simulink model "Miss_Sim_MatrixPilot"  (Simulink 7.0)
settings: Solver=ode1  SolverMode=SingleTasking  StartTime=0.0  StopTime=120  FixedStep=0.00025  MaxStep=0.01  MinStep=0.000001  RelTol=1e-12  AbsTol=1e-12
values from neighbouring files (symbols this model uses):
  alpha = [-180.     -90.        -5.         0.         5.        10.        15.        90.       180.       ]    [Miss_Data.m]
  Bref = 1.4    [Miss_Data.m]
  Clail = [ 0.         0.         0.         0.         0.         0.         0.         0.         0.       ]    [Miss_Data.m]
  Clp = [-0.5000    -0.5000    -0.496303  -0.494610  -0.492441  -0.492625  -0.522141  -0.5000    -0.5000   ]    [Miss_Data.m]
  Clr = [ 0.         0.         0.064175   0.123689   0.182593   0.241565   0.304725   0.         0.       ]    [Miss_Data.m]
  Clrud = [-0.000045  -0.000045  -0.000051  -0.000049  -0.000047  -0.000043  -0.000039  -0.000045  -0.000045 ]    [Miss_Data.m]
  Clv = [ 0.         0.        -0.098934  -0.137639  -0.176627  -0.217863  -0.281334   0.         0.       ]    [Miss_Data.m]
  Cmele = [-0.0180    -0.0180    -0.019125  -0.019236  -0.019052  -0.018576  -0.017796  -0.0180    -0.0180   ]    [Miss_Data.m]
  Cmq = [-12.3     -12.3      -12.288971 -12.358734 -12.331396 -12.223111 -12.072741 -12.3      -12.3      ]    [Miss_Data.m]
  Cmtot = [ 0.         2.         0.097340   0.036740  -0.047230  -0.137480  -0.110880  -2.         0.       ]    [Miss_Data.m]
  Cnail = [ 0.         0.         0.         0.         0.         0.         0.         0.         0.       ]    [Miss_Data.m]
  Cnp = [ 0.         0.         0.027830  -0.031473  -0.087981  -0.137950  -0.158851   0.         0.       ]    [Miss_Data.m]
  Cnr = [ 0.         0.        -0.041684  -0.040009  -0.043373  -0.056062  -0.120565   0.         0.       ]    [Miss_Data.m]
  Cnrud = [ 0.         0.         0.000628   0.000668   0.000698   0.000717   0.000725   0.         0.       ]    [Miss_Data.m]
  Cnv = [ 0.         0.         0.011072   0.000612  -0.009401  -0.018785  -0.019172   0.         0.       ]    [Miss_Data.m]
  Cref = 0.20    (= 0.2)    [Miss_Data.m]
  CROSS_TRACK = 1    [MatrixPilot_Parameters.m]
  CXq = [ 0.         0.        -0.507981  -0.147630   0.201483   0.570203   1.026474   0.         0.       ]    [Miss_Data.m]
  CXtot = [ 0.03       0.        -0.060470  -0.054540   0.003010   0.075240  -0.109550   0.         0.03     ]    [Miss_Data.m]
  CYp = [ 0.         0.        -0.217329  -0.145848  -0.074905  -0.009210   0.015572   0.         0.       ]    [Miss_Data.m]
  CYr = [ 0.         0.         0.049134   0.076782   0.103755   0.129584   0.152004   0.         0.       ]    [Miss_Data.m]
  CYrud = [-0.0016    -0.0016    -0.001484  -0.001575  -0.001641  -0.001681  -0.001693  -0.0016    -0.0016   ]    [Miss_Data.m]
  CYv = [ 0.         0.        -0.204296  -0.201289  -0.208918  -0.263073  -0.644029   0.         0.       ]    [Miss_Data.m]
  CZele = [-0.0067    -0.0067    -0.006924  -0.006962  -0.006897  -0.006734  -0.006498  -0.0067    -0.0067   ]    [Miss_Data.m]
  CZq = [ 0.         0.        -9.116849  -8.745556  -8.332987  -7.894125  -7.541102   0.         0.       ]    [Miss_Data.m]
  CZtot = [ 0.        10.         0.102580  -0.382550  -0.864940  -1.339340  -1.876430 -10.         0.       ]    [Miss_Data.m]
  DH = 10.    (= 10)    [MatrixPilot_Parameters.m]
  ele_damping = 0.7    [Miss_Data.m]
  ele_def_max = 30.    (= 30)    [Miss_Data.m]
  ele_frequency = 150.    (= 150)    [Miss_Data.m]
  ele_rate_limit = 285.    (= 285)    [Miss_Data.m]
  Ixx = 0.03004    [Miss_Data.m]
  Ixy = 0.    (= 0)    [Miss_Data.m]
  Ixz = 0.00137    [Miss_Data.m]
  Iyx = Ixy    (= 0)    [Miss_Data.m]
  Iyy = 0.01916    [Miss_Data.m]
  Iyz = 0.    (= 0)    [Miss_Data.m]
  Izx = Ixz    (= 0.00137)    [Miss_Data.m]
  Izy = Iyz    (= 0)    [Miss_Data.m]
  Izz = 0.04573    [Miss_Data.m]
  Mass = 0.950    (= 0.95)    [Miss_Data.m]
  rud_damping = 0.7    [Miss_Data.m]
  rud_def_max = 30.    (= 30)    [Miss_Data.m]
  rud_frequency = 150.    (= 150)    [Miss_Data.m]
  rud_rate_limit = 285.    (= 285)    [Miss_Data.m]
  SPEED_CONTROL = 1    [MatrixPilot_Parameters.m]
  Sref = 0.28    [Miss_Data.m]
  T_max = 1.    (= 1)    [MatrixPilot_Parameters.m]
  T_min = 0.35    [MatrixPilot_Parameters.m]
  Tdgps = 1.    (= 1)    [Miss_Data.m]
  theta_0 = -15.    (= -15)    [MatrixPilot_Parameters.m]
  theta_max = 15.    (= 15)    [MatrixPilot_Parameters.m]
  theta_min = -15.    (= -15)    [MatrixPilot_Parameters.m]
  Tmax = 10.    (= 10)    [Miss_Data.m]
  Vsp = 10.    (= 10)    [MatrixPilot_Parameters.m]
  WAYPOINT_RADIUS = 30.    (= 30)    [MatrixPilot_Parameters.m]
undefined symbols (not defined in the file or in its folder): F, MIL, Moderate
libraries: simulink x41, simulink_extras x26, dspstat3 x2, aerospace x1, aerolibanim x1, aerolibwind2 x1
(part 1 of 2)
settings Model: Creator=bizard  LastModifiedBy=bizard
settings SolverCC: InitialStep=0.000001  AutoInsertRateTranBlk=on
settings OptimizationCC: BooleanDataType=off
settings DebuggingCC: SaveWithParameterizedLinksMsg=none  SignalResolutionControl=TryResolveAllWithWarning  SolverPrmCheckMsg=none  MultiTaskDSMMsg=warning  MultiTaskCondExecSysMsg=none  StrictBusMsg=None
settings HardwareCC: TargetEndianess=LittleEndian  TargetHWDeviceType=MATLAB Host  ProdEqTarget=off
settings RTWCC: IncludeERTFirstTime=on

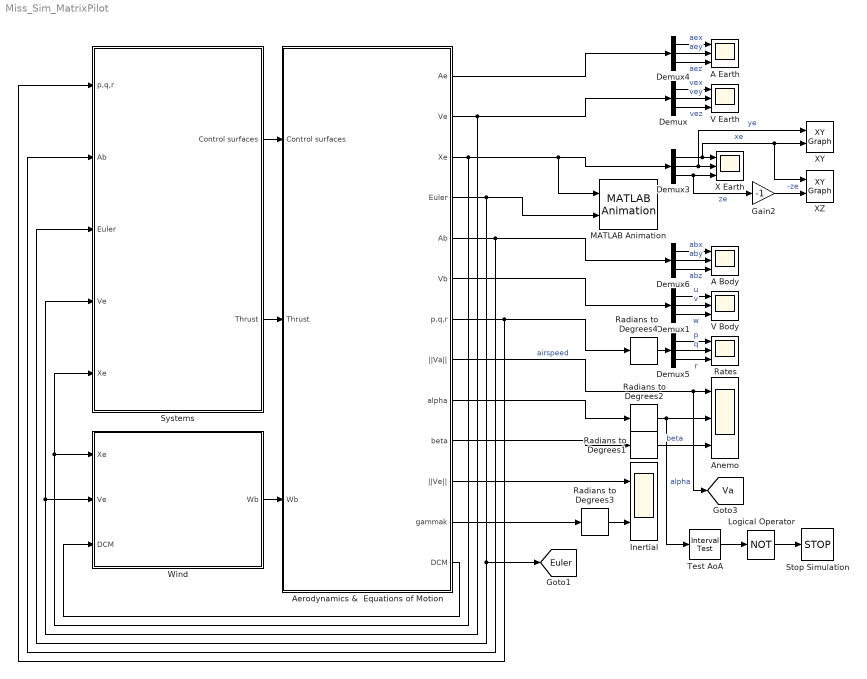
== system Miss_Sim_MatrixPilot ==
  A Body : Scope  NumInputPorts=3
      settings: TimeRange=300  YMin=0~-0.1~0  YMax=30~0.1~2  SaveName=ScopeData3  MaxDataPoints=60000  Decimation=10
  A Earth : Scope  NumInputPorts=3
      settings: TimeRange=60  YMin=-10~-10~-4  YMax=10~10~8  MaxDataPoints=600000  Decimation=10
  Aerodynamics &  Equations of Motion : Subsystem
  Anemo : Scope  NumInputPorts=3
      settings: TimeRange=20  YMin=8.7~0~-8  YMax=10.3~5~8  SaveName=ScopeData6  MaxDataPoints=600000  Decimation=10
  Demux{,1,3..6} (6 alike) : Demux  Outputs=3
  Gain2 : Gain  Gain=-1  SaturateOnIntegerOverflow=on
  Inertial : Scope  NumInputPorts=2
      settings: TimeRange=50  YMin=7.5~-10  YMax=10.5~-0  SaveName=ScopeData7  MaxDataPoints=600000  Decimation=10
  Logical Operator : Logic  Operator=NOT  AllPortsSameDT=off  OutDataTypeMode=boolean
  MATLAB Animation : aerolibanim/MATLAB Animation  Vehicles=1  Geometries='astredwedge.mat'  BoundingBoxCoordinates=[-50,50,-50,50,-50,50]  CameraOffset=[-150,-50,0]  CameraViewAngle=3  SampleTime=0.1  FigurePosition=[1080,494,275,214]
  Radians to Degrees{1..4} (4 alike) : simulink_extras/Transformations/Radians to Degrees  SystemSampleTime=-1
  Rates : Scope  NumInputPorts=3
      settings: YMin=-100~-100~-100  YMax=100~100~100  MaxDataPoints=600000  Decimation=10
  Stop Simulation : Stop
  Systems : Subsystem
  Test AoA : simulink/Logic and Bit Operations/Interval Test  SystemSampleTime=-1  IntervalClosedRight=on  uplimit=15  IntervalClosedLeft=on  lowlimit=-15  LogicOutDataTypeMode=boolean
  V Body : Scope  NumInputPorts=3
      settings: TimeRange=300  YMin=0~-0.1~0  YMax=30~0.1~2  SaveName=ScopeData4  MaxDataPoints=60000  Decimation=10
  V Earth : Scope  NumInputPorts=3
      settings: TimeRange=60  YMin=-15~-15~-3  YMax=10~15~2  SaveName=ScopeData2  MaxDataPoints=600000  Decimation=10  SampleInput=on
  Wind : Subsystem
  X Earth : Scope  NumInputPorts=3
      settings: TimeRange=60  YMin=-150~-100~-80  YMax=150~100~-45  SaveName=ScopeData9  MaxDataPoints=600000  Decimation=10
  XY : simulink/Sinks/XY Graph  SystemSampleTime=-1  xmin=-150  xmax=150  ymin=-150  ymax=150  st=.1
  XZ : simulink/Sinks/XY Graph  SystemSampleTime=-1  xmin=-150  xmax=150  ymin=0  ymax=100  st=.1
  tag scope: Euler=global, Va=global
  wires:
  Aerodynamics &  Equations of Motion/9(alpha) -> Radians to Degrees2/1
  Aerodynamics &  Equations of Motion/10(beta) -> Radians to Degrees1/1
  Radians to Degrees1/1 -> Anemo/3  "beta"
  Demux1/1 -> V Body/1  "u"
  Demux1/2 -> V Body/2  "v"
  Demux1/3 -> V Body/3  "w"
  Radians to Degrees2/1 -> Anemo/2, Test AoA/1  "alpha"
  Aerodynamics &  Equations of Motion/8(||Va||) -> Anemo/1, [Va]  "airspeed"
  Demux5/1 -> Rates/1  "p"
  Demux5/2 -> Rates/2  "q"
  Demux5/3 -> Rates/3  "r"
  Radians to Degrees4/1 -> Demux5/1
  Aerodynamics &  Equations of Motion/7(p,q,r) -> Radians to Degrees4/1, Systems/1(p,q,r)
  Aerodynamics &  Equations of Motion/6(Vb) -> Demux1/1
  Aerodynamics &  Equations of Motion/4(Euler) -> MATLAB Animation/2, Systems/3(Euler), [Euler]
  Demux/1 -> V Earth/1  "vex"
  Demux/2 -> V Earth/2  "vey"
  Demux/3 -> V Earth/3  "vez"
  Gain2/1 -> XZ/2  "-ze"
  Aerodynamics &  Equations of Motion/3(Xe) -> Demux3/1, MATLAB Animation/1, Systems/5(Xe), Wind/1(Xe)
  Aerodynamics &  Equations of Motion/2(Ve) -> Systems/4(Ve), Wind/2(Ve), Demux/1
  Systems/2(Thrust) -> Aerodynamics &  Equations of Motion/2(Thrust)
  Systems/1(Control surfaces) -> Aerodynamics &  Equations of Motion/1(Control surfaces)
  Aerodynamics &  Equations of Motion/1(Ae) -> Demux4/1
  Demux4/3 -> A Earth/3  "aez"
  Demux4/2 -> A Earth/2  "aey"
  Demux4/1 -> A Earth/1  "aex"
  Demux6/1 -> A Body/1  "abx"
  Demux6/3 -> A Body/3  "abz"
  Aerodynamics &  Equations of Motion/5(Ab) -> Demux6/1, Systems/2(Ab)
  Wind/1(Wb) -> Aerodynamics &  Equations of Motion/3(Wb)
  Demux6/2 -> A Body/2  "aby"
  Test AoA/1 -> Logical Operator/1
  Logical Operator/1 -> Stop Simulation/1
  Aerodynamics &  Equations of Motion/11(||Ve||) -> Inertial/1
  Aerodynamics &  Equations of Motion/13(DCM) -> Wind/3(DCM)
  Demux3/1 -> X Earth/1, XY/2, XZ/1  "xe"
  Demux3/2 -> X Earth/2, XY/1  "ye"
  Demux3/3 -> X Earth/3, Gain2/1  "ze"
  Aerodynamics &  Equations of Motion/12(gammak) -> Radians to Degrees3/1
  Radians to Degrees3/1 -> Inertial/2

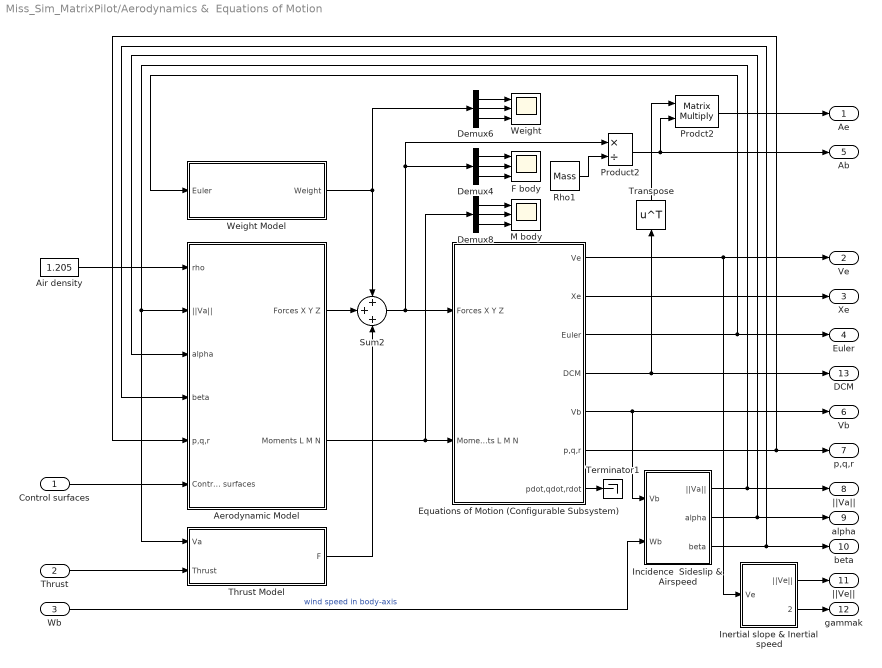
== system Miss_Sim_MatrixPilot/Aerodynamics &  Equations of Motion ==
  Control surfaces : Inport
  Thrust : Inport  Port=2
  Wb : Inport  Port=3
  Aerodynamic Model : Subsystem
  Air density : Constant  Value=1.205
  Demux4 : Demux  Outputs=3
  Demux6 : Demux  Outputs=3
  Demux8 : Demux  Outputs=3
  Equations of Motion (Configurable Subsystem) : Subsystem  BlockChoice=Quaternions
      link override Euler Angles: Inertia=[Ixx Ixy Ixz ; Iyx Iyy Iyz ; Izx Izy Izz]  eul_0="[0.    0.    0.]"  Vm_0="[25.   0.   0.]"  Mass=Mass  xme_0=[0. 0. 0.]
      link override Quaternions: Inertia="[Ixx  -Ixy  -Ixz;  -Iyx  Iyy  -Iyz;  -Izx  -Izy  Izz]"  Mass=Mass  Vm_0=[10 0 0]  eul_0=[0 0. 0]  xme_0=[0 0 -75.]
      settings: AttributesFormatString=%<BlockChoice>  MemberBlocks=Euler Angles,Quaternions
      settings: TemplateBlock=|
      | aerospace/6DoF/Equations of Motion
      | (Configurable Subsystem)
  F body : Scope  NumInputPorts=3
      settings: YMin=-20~-1~-100  YMax=27.5~1~10  SaveName=ScopeData5  MaxDataPoints=600000  Decimation=10
  Incidence  Sideslip & Airspeed : Subsystem
  Inertial slope & Inertial speed : Subsystem
  M body : Scope  NumInputPorts=3
      settings: TimeRange=300  YMin=13~-1~-2.5  YMax=20.5~1~1.5  SaveName=ScopeData10  MaxDataPoints=600000  Decimation=10
  Prodct2 : Product  Multiplication=Matrix(*)  SaturateOnIntegerOverflow=on  RndMeth=Zero  InputSameDT=on
  Product2 : Product  Inputs=*/  SaturateOnIntegerOverflow=on  RndMeth=Zero  InputSameDT=on
  Rho1 : Constant  Value=Mass
  Sum2 : Sum  Inputs=+++  SaturateOnIntegerOverflow=on  InputSameDT=on
  Terminator1 : Terminator
  Thrust Model : Subsystem
  Transpose : Math  Orientation=up  Operator=transpose  SaturateOnIntegerOverflow=on
  "Weight " : Scope  NumInputPorts=3
      settings: TimeRange=300  YMin=13~-1~0  YMax=20.5~1~50  SaveName=ScopeData8  MaxDataPoints=600000  Decimation=10
  Weight Model : Subsystem
  Ae : Outport
  Ve : Outport  Port=2
  Xe : Outport  Port=3
  Euler : Outport  Port=4
  Ab : Outport  Port=5
  Vb : Outport  Port=6
  p,q,r : Outport  Port=7
  ||Va|| : Outport  Port=8
  alpha : Outport  Port=9
  beta : Outport  Port=10
  ||Ve|| : Outport  Port=11
  gammak : Outport  Port=12
  DCM : Outport  Port=13
  wires:
  Equations of Motion (Configurable Subsystem)/7(pdot,qdot,rdot) -> Terminator1/1
  Equations of Motion (Configurable Subsystem)/1(Ve) -> Inertial slope & Inertial speed/1(Ve), Ve/1
  Equations of Motion (Configurable Subsystem)/3(Euler) -> Weight Model/1(Euler), Euler/1
  Equations of Motion (Configurable Subsystem)/5(Vb) -> Incidence  Sideslip & Airspeed/1(Vb), Vb/1
  Incidence  Sideslip & Airspeed/2(alpha) -> alpha/1, Aerodynamic Model/3(alpha)
  Equations of Motion (Configurable Subsystem)/6(p,q,r) -> p,q,r/1, Aerodynamic Model/5(p,q,r)
  Incidence  Sideslip & Airspeed/3(beta) -> beta/1, Aerodynamic Model/4(beta)
  Incidence  Sideslip & Airspeed/1(||Va||) -> ||Va||/1, Aerodynamic Model/2(||Va||), Thrust Model/1(Va)
  Equations of Motion (Configurable Subsystem)/2(Xe) -> Xe/1
  Thrust Model/1(F) -> Sum2/3
  Weight Model/1(Weight) -> Sum2/1, Demux6/1
  Demux4/1 -> F body/1
  Demux4/2 -> F body/2
  Demux4/3 -> F body/3
  Aerodynamic Model/1(Forces X Y Z) -> Sum2/2
  Sum2/1 -> Equations of Motion (Configurable Subsystem)/1(Forces X Y Z), Demux4/1, Product2/1
  Inertial slope & Inertial speed/1(||Ve||) -> ||Ve||/1
  Inertial slope & Inertial speed/2(gammak) -> gammak/1
  Demux6/1 -> "Weight "/1
  Demux6/2 -> "Weight "/2
  Demux6/3 -> "Weight "/3
  Demux8/1 -> M body/1
  Demux8/2 -> M body/2
  Demux8/3 -> M body/3
  Aerodynamic Model/2(Moments L M N) -> Demux8/1, Equations of Motion (Configurable Subsystem)/2(Moments L M N)
  Control surfaces/1 -> Aerodynamic Model/6(Control surfaces)
  Thrust/1 -> Thrust Model/2(Thrust)
  Product2/1 -> Ab/1, Prodct2/2
  Equations of Motion (Configurable Subsystem)/4(DCM) -> Transpose/1, DCM/1
  Transpose/1 -> Prodct2/1
  Prodct2/1 -> Ae/1
  Wb/1 -> Incidence  Sideslip & Airspeed/2(Wb)  "wind speed in body-axis"
  Rho1/1 -> Product2/2
  Air density/1 -> Aerodynamic Model/1(rho)

== system Miss_Sim_MatrixPilot/Systems ==
  p,q,r : Inport
  Ab : Inport  Port=2
  Euler : Inport  Port=3
  Ve : Inport  Port=4
  Xe : Inport  Port=5
  Actuators : Subsystem
  Data processing : Subsystem
  NGC : Subsystem
  Sensors : Subsystem
  Control surfaces : Outport
  Thrust : Outport  Port=2
  wires:
  NGC/1(rudc) -> Actuators/1(rudc)
  NGC/2(elec) -> Actuators/2(elec)
  Actuators/1(Control surfaces) -> Control surfaces/1
  Actuators/2(Thrust) -> Thrust/1
  NGC/3(Tc) -> Actuators/3(Tc)
  p,q,r/1 -> Sensors/1(p,q,r)
  Xe/1 -> Sensors/5(Xe)
  Ve/1 -> Sensors/4(Ve)
  Euler/1 -> Sensors/3(Euler)
  Ab/1 -> Sensors/2(Ab)
  Data processing/4(||Va||) -> NGC/4(||Va||)
  Data processing/1(DCM) -> NGC/1(DCM)
  Data processing/2(We) -> NGC/2(We)
  Sensors/2(GPS) -> Data processing/2(GPS)
  Data processing/3(Vaxy) -> NGC/3(Vaxy)
  Sensors/1(Acc) -> Data processing/1(Acc)
  Sensors/3("p,q,r ") -> Data processing/3(p,q,r), NGC/7(p,q,r)
  Data processing/6(Ve) -> NGC/6(Ve)
  Data processing/5(Xe) -> NGC/5(Xe)

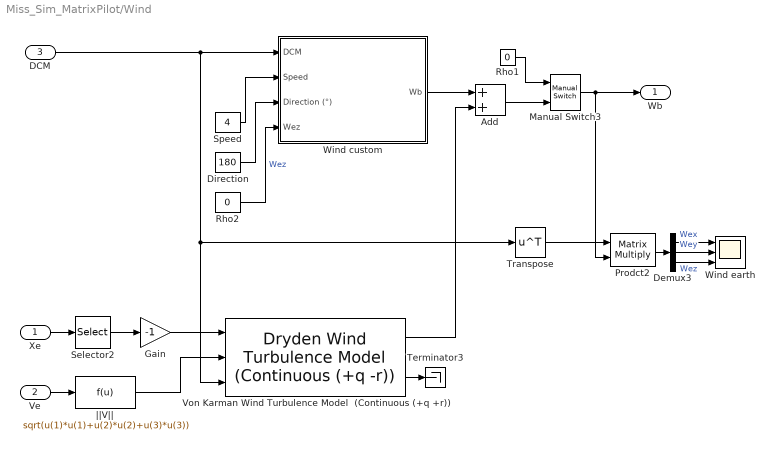
== system Miss_Sim_MatrixPilot/Wind ==
  Xe : Inport
  Ve : Inport  Port=2
  DCM : Inport  Port=3
  Add : Sum  OutDataType=sfix(16)  OutScaling=2^-10
  Demux3 : Demux  Outputs=3
  Direction : Constant  Value=180
  Gain : Gain  Gain=-1  ParameterDataType=sfix(16)  ParameterScaling=2^0  OutDataType=sfix(16)  OutScaling=2^0
  Manual Switch3 : simulink/Signal Routing/Manual Switch  SystemSampleTime=-1  sw=1  action=0  varsize=off
  Prodct2 : Product  Multiplication=Matrix(*)  SaturateOnIntegerOverflow=on  RndMeth=Zero  InputSameDT=on
  Rho1 : Constant  Value=0  VectorParams1D=off
  Rho2 : Constant  Value=0
  Selector2 : Selector  InputPortWidth=3  IndexOptions=Index vector (dialog)  Indices=[3]  OutputSizes=1
  Speed : Constant  Value=4
  Terminator3 : Terminator
  Transpose : Math  Operator=transpose  SaturateOnIntegerOverflow=on
  Von Karman Wind Turbulence Model  (Continuous (+q +r)) : aerolibwind2/Dryden Wind Turbulence Model  (Continuous (+q -r))  SystemSampleTime=-1  units=Metric (MKS)  spec=MIL-F-8785C  model=Continuous Dryden (-q +r)  W20=4  Wdeg=180  TurbProb=10^-3 - Moderate  L_high=762  Wingspan=1.4  ts=1  Seed=[23341 23342 23343 23344]  T_on=on
  Wind custom : Subsystem
  Wind earth : Scope  NumInputPorts=3
      settings: TimeRange=60  YMin=-1~-1~-1  YMax=1~1~1  SaveName=ScopeData33  MaxDataPoints=600000  Decimation=100
  ||V|| : Fcn  Expr=sqrt(u(1)*u(1)+u(2)*u(2)+u(3)*u(3))
  Wb : Outport
  wires:
  Direction/1 -> Wind custom/3(Direction (°))
  Speed/1 -> Wind custom/2(Speed)
  Rho2/1 -> Wind custom/4(Wez)  "Wez"
  DCM/1 -> Wind custom/1(DCM), Von Karman Wind Turbulence Model  (Continuous (+q +r))/3, Transpose/1
  Ve/1 -> ||V||/1
  Xe/1 -> Selector2/1
  ||V||/1 -> Von Karman Wind Turbulence Model  (Continuous (+q +r))/2
  Gain/1 -> Von Karman Wind Turbulence Model  (Continuous (+q +r))/1
  Wind custom/1(Wb) -> Add/1
  Add/1 -> Manual Switch3/2
  Von Karman Wind Turbulence Model  (Continuous (+q +r))/1 -> Add/2
  Von Karman Wind Turbulence Model  (Continuous (+q +r))/2 -> Terminator3/1
  Demux3/1 -> Wind earth/1  "Wex"
  Demux3/2 -> Wind earth/2  "Wey"
  Demux3/3 -> Wind earth/3  "Wez"
  Prodct2/1 -> Demux3/1
  Transpose/1 -> Prodct2/1
  Rho1/1 -> Manual Switch3/1
  Manual Switch3/1 -> Wb/1, Prodct2/2
  Selector2/1 -> Gain/1

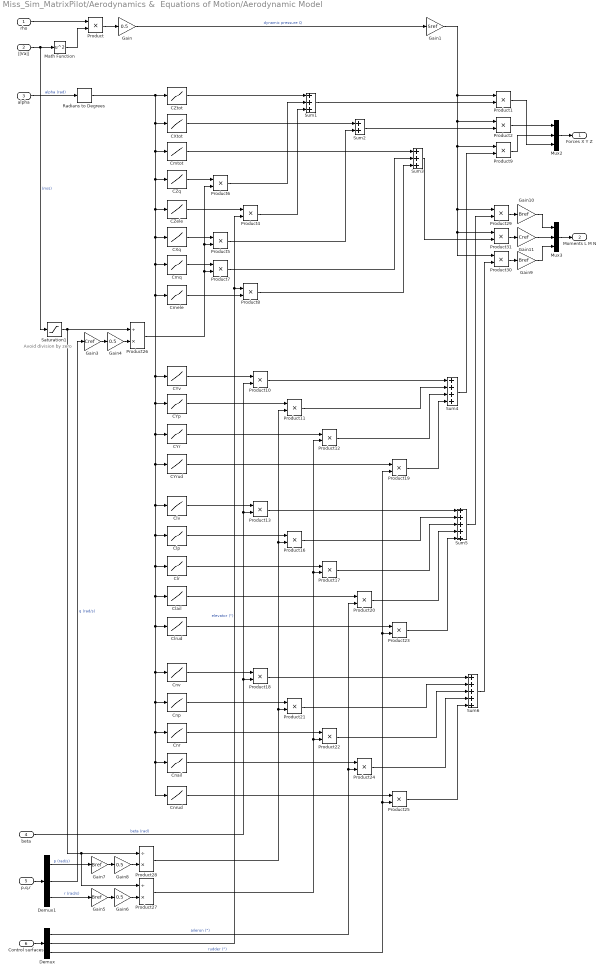
== system Miss_Sim_MatrixPilot/Aerodynamics &  Equations of Motion/Aerodynamic Model ==
  note: Avoid division
      | by zero
  rho : Inport
  ||Va|| : Inport  Port=2
  alpha : Inport  Port=3
  beta : Inport  Port=4
  p,q,r : Inport  Port=5
  Control surfaces : Inport  Port=6
  CXq : Lookup  InputValues=alpha  Table=CXq  SaturateOnIntegerOverflow=on
  CXtot : Lookup  InputValues=alpha  Table=CXtot  SaturateOnIntegerOverflow=on
  CYp : Lookup  InputValues=alpha  Table=CYp  SaturateOnIntegerOverflow=on
  CYr : Lookup  InputValues=alpha  Table=CYr  SaturateOnIntegerOverflow=on
  CYrud : Lookup  InputValues=alpha  Table=CYrud  SaturateOnIntegerOverflow=on
  CYv : Lookup  InputValues=alpha  Table=CYv  SaturateOnIntegerOverflow=on
  CZele : Lookup  InputValues=alpha  Table=CZele  SaturateOnIntegerOverflow=on
  CZq : Lookup  InputValues=alpha  Table=CZq  SaturateOnIntegerOverflow=on
  CZtot : Lookup  InputValues=alpha  Table=CZtot  SaturateOnIntegerOverflow=on
  Clail : Lookup  InputValues=alpha  Table=Clail  SaturateOnIntegerOverflow=on
  Clp : Lookup  InputValues=alpha  Table=Clp  SaturateOnIntegerOverflow=on
  Clr : Lookup  InputValues=alpha  Table=Clr  SaturateOnIntegerOverflow=on
  Clrud : Lookup  InputValues=alpha  Table=Clrud  SaturateOnIntegerOverflow=on
  Clv : Lookup  InputValues=alpha  Table=Clv  SaturateOnIntegerOverflow=on
  Cmele : Lookup  InputValues=alpha  Table=Cmele  SaturateOnIntegerOverflow=on
  Cmq : Lookup  InputValues=alpha  Table=Cmq  SaturateOnIntegerOverflow=on
  Cmtot : Lookup  InputValues=alpha  Table=Cmtot  SaturateOnIntegerOverflow=on
  Cnail : Lookup  InputValues=alpha  Table=Cnail  SaturateOnIntegerOverflow=on
  Cnp : Lookup  InputValues=alpha  Table=Cnp  SaturateOnIntegerOverflow=on
  Cnr : Lookup  InputValues=alpha  Table=Cnr  SaturateOnIntegerOverflow=on
  Cnrud : Lookup  InputValues=alpha  Table=Cnrud  SaturateOnIntegerOverflow=on
  Cnv : Lookup  InputValues=alpha  Table=Cnv  SaturateOnIntegerOverflow=on
  Demux : Demux  Outputs=3
  Demux1 : Demux  Outputs=3
  Gain{,4,6,8} (4 alike) : Gain  Gain=0.5  SaturateOnIntegerOverflow=on
  Gain1 : Gain  Gain=Sref  SaturateOnIntegerOverflow=on
  Gain{5,7,9..10} (4 alike) : Gain  Gain=Bref  SaturateOnIntegerOverflow=on
  Gain11 : Gain  Gain=Cref  SaturateOnIntegerOverflow=on
  Gain3 : Gain  Gain=Cref  SaturateOnIntegerOverflow=on
  Math Function : Math  Operator=square  SaturateOnIntegerOverflow=on
  Mux2 : Mux  Inputs=3
  Mux3 : Mux  Inputs=3
  Product{,1..2,4..13,16..25,29..31} (26 alike) : Product  SaturateOnIntegerOverflow=on  RndMeth=Zero  InputSameDT=on
  Product26 : Product  Inputs=/*  SaturateOnIntegerOverflow=on  RndMeth=Zero  InputSameDT=on
  Product27 : Product  Inputs=/*  SaturateOnIntegerOverflow=on  RndMeth=Zero  InputSameDT=on
  Product28 : Product  Inputs=/*  SaturateOnIntegerOverflow=on  RndMeth=Zero  InputSameDT=on
  Radians to Degrees : simulink_extras/Transformations/Radians to Degrees  SystemSampleTime=-1
  Saturation1 : Saturate  UpperLimit=1000000  LowerLimit=0.001
  Sum1 : Sum  Inputs=+++  InputSameDT=on
  Sum2 : Sum  SaturateOnIntegerOverflow=on  InputSameDT=on
  Sum3 : Sum  Inputs=+++  SaturateOnIntegerOverflow=on  InputSameDT=on
  Sum4 : Sum  Inputs=++++  SaturateOnIntegerOverflow=on  InputSameDT=on
  Sum5 : Sum  Inputs=+++++  SaturateOnIntegerOverflow=on  InputSameDT=on
  Sum6 : Sum  Inputs=+++++  SaturateOnIntegerOverflow=on  InputSameDT=on
  Forces X Y Z : Outport
  Moments L M N : Outport  Port=2
  wires:
  Mux2/1 -> Forces X Y Z/1
  alpha/1 -> Radians to Degrees/1  "alpha (rad)"
  Radians to Degrees/1 -> CZtot/1, Cmtot/1, CZq/1, CZele/1, Cmq/1, CYv/1, CYp/1, CYr/1, Clv/1, Clr/1, Clail/1, Cnv/1, Cnp/1, Cnr/1, Cnail/1, Cnrud/1, Clrud/1, Clp/1, CYrud/1, Cmele/1, CXq/1, CXtot/1
  rho/1 -> Product/1
  Math Function/1 -> Product/2
  Product/1 -> Gain/1
  Gain/1 -> Gain1/1  "dynamic pressure Q"
  Gain1/1 -> Product1/1, Product2/1, Product9/1, Product30/1, Product31/1, Product29/1
  Product1/1 -> Mux2/3
  CZtot/1 -> Sum1/1
  Sum1/1 -> Product1/2
  CZele/1 -> Product4/1
  Control surfaces/1 -> Demux/1
  Demux/2 -> Product4/2, Product8/1  "elevator (°)"
  Product4/1 -> Sum1/3
  p,q,r/1 -> Demux1/1
  CXq/1 -> Product5/1
  Demux1/2 -> Gain3/1  "q (rad/s)"
  CXtot/1 -> Sum2/1
  Sum2/1 -> Product2/2
  Product5/1 -> Sum2/2
  Cmq/1 -> Product7/1
  Cmtot/1 -> Sum3/1
  Sum3/1 -> Product31/2
  Product7/1 -> Sum3/2
  Cmele/1 -> Product8/2
  beta/1 -> Product10/2, Product13/2, Product18/2  "beta (rad)"
  Product9/1 -> Mux2/2
  Sum4/1 -> Product9/2
  CYv/1 -> Product10/1
  Product10/1 -> Sum4/1
  CYp/1 -> Product11/1
  Product11/1 -> Sum4/2
  CYr/1 -> Product12/1
  Product12/1 -> Sum4/3
  Clv/1 -> Product13/1
  Product13/1 -> Sum5/1
  Sum5/1 -> Product29/2
  Clp/1 -> Product16/1
  Product16/1 -> Sum5/2
  Clr/1 -> Product17/1
  Product17/1 -> Sum5/3
  Cnv/1 -> Product18/1
  Product18/1 -> Sum6/1
  Sum6/1 -> Product30/2
  Product8/1 -> Sum3/3
  Product19/1 -> Sum4/4
  CYrud/1 -> Product19/1
  Demux/3 -> Product19/2, Product23/2, Product25/2  "rudder (°)"
  Clail/1 -> Product20/1
  Product20/1 -> Sum5/4
  Demux/1 -> Product20/2, Product24/2  "aileron (°)"
  Cnp/1 -> Product21/1
  Product21/1 -> Sum6/2
  Cnr/1 -> Product22/1
  Product22/1 -> Sum6/3
  Clrud/1 -> Product23/1
  Product23/1 -> Sum5/5
  Cnail/1 -> Product24/1
  Product24/1 -> Sum6/4
  Cnrud/1 -> Product25/1
  Product25/1 -> Sum6/5
  Product2/1 -> Mux2/1
  Product6/1 -> Sum1/2
  CZq/1 -> Product6/1
  Gain3/1 -> Gain4/1
  Gain4/1 -> Product26/2
  Product26/1 -> Product6/2, Product5/2, Product7/2
  Saturation1/1 -> Product26/1, Product28/1, Product27/1
  Gain5/1 -> Gain6/1
  Gain6/1 -> Product27/2
  Gain7/1 -> Gain8/1
  Gain8/1 -> Product28/2
  Demux1/1 -> Gain7/1  "p (rad/s)"
  Product28/1 -> Product11/2, Product16/2, Product21/2
  Demux1/3 -> Gain5/1  "r (rad/s)"
  Product27/1 -> Product12/2, Product17/2, Product22/2
  Mux3/1 -> Moments L M N/1
  Product31/1 -> Gain11/1
  Product29/1 -> Gain10/1
  Product30/1 -> Gain9/1
  Gain11/1 -> Mux3/2
  Gain10/1 -> Mux3/1
  Gain9/1 -> Mux3/3
  ||Va||/1 -> Math Function/1, Saturation1/1  "(m/s)"

== system Miss_Sim_MatrixPilot/Aerodynamics &  Equations of Motion/Equations of Motion (Configurable Subsystem) ==
  Forces X Y Z : Inport  OutDataType=sfix(16)  OutScaling=2^0
  Moments L M N : Inport  Port=2  OutDataType=sfix(16)  OutScaling=2^0
  Quaternions : aerospace/6DoF/Quaternions  SystemSampleTime=-1  xme_0=[0 0 -75.]  Vm_0=[10 0 0]  eul_0=[0 0. 0]  pm_0=[0 0 0]  Mass=Mass  Inertia="[Ixx  -Ixy  -Ixz;  -Iyx  Iyy  -Iyz;  -Izx  -Izy  Izz]"
  Ve : Outport  OutDataType=sfix(16)  OutScaling=2^0
  Xe : Outport  Port=2  OutDataType=sfix(16)  OutScaling=2^0
  Euler : Outport  Port=3  OutDataType=sfix(16)  OutScaling=2^0
  DCM : Outport  Port=4  OutDataType=sfix(16)  OutScaling=2^0
  Vb : Outport  Port=5  OutDataType=sfix(16)  OutScaling=2^0
  p,q,r : Outport  Port=6  OutDataType=sfix(16)  OutScaling=2^0
  pdot,qdot,rdot : Outport  Port=7  OutDataType=sfix(16)  OutScaling=2^0
  wires:
  Forces X Y Z/1 -> Quaternions/1
  Moments L M N/1 -> Quaternions/2
  Quaternions/1 -> Ve/1
  Quaternions/2 -> Xe/1
  Quaternions/3 -> Euler/1
  Quaternions/4 -> DCM/1
  Quaternions/5 -> Vb/1
  Quaternions/6 -> p,q,r/1
  Quaternions/7 -> pdot,qdot,rdot/1

== system Miss_Sim_MatrixPilot/Aerodynamics &  Equations of Motion/Incidence  Sideslip & Airspeed ==
  note: Avoid division
      | by zero
  Vb : Inport
  Wb : Inport  Port=2
  Demux2 : Demux  Outputs=3
  Mux : Mux  Inputs=2
  Mux1 : Mux  Inputs=2
  Saturation1 : Saturate  UpperLimit=1000  LowerLimit=0.01
  Saturation2 : Saturate  UpperLimit=1000  LowerLimit=0.01
  Sum2 : Sum  Inputs=+-  SaturateOnIntegerOverflow=on  InputSameDT=on
  asin(v/V) : Fcn  Expr=asin(u[2]/u[1])
  atan(w/u) : Fcn  Expr=atan2(u[2],u[1])
  ||V|| : Fcn  Expr=sqrt(u(1)*u(1)+u(2)*u(2)+u(3)*u(3))
  ||Va|| : Outport
  alpha : Outport  Port=2
  beta : Outport  Port=3
  wires:
  ||V||/1 -> ||Va||/1, Saturation1/1
  atan(w/u)/1 -> alpha/1
  Mux/1 -> asin(v/V)/1
  asin(v/V)/1 -> beta/1
  Demux2/1 -> Saturation2/1
  Demux2/3 -> Mux1/2
  Demux2/2 -> Mux/2
  Mux1/1 -> atan(w/u)/1
  Saturation2/1 -> Mux1/1
  Saturation1/1 -> Mux/1
  Vb/1 -> Sum2/1
  Sum2/1 -> Demux2/1, ||V||/1
  Wb/1 -> Sum2/2  "wind speed in body-axis"

== system Miss_Sim_MatrixPilot/Aerodynamics &  Equations of Motion/Inertial slope & Inertial speed ==
  Ve : Inport
  Demux2 : Demux  Outputs=3
  Mux : Mux  Inputs=2
  Saturation1 : Saturate  UpperLimit=1000  LowerLimit=0.1
  Terminator1 : Terminator
  Terminator2 : Terminator
  asin(vz/Ve) : Fcn  Expr=-asin(u[2]/u[1])
  ||V|| : Fcn  Expr=sqrt(u(1)*u(1)+u(2)*u(2)+u(3)*u(3))
  ||Ve|| : Outport
  gammak : Outport  Port=2
  wires:
  ||V||/1 -> ||Ve||/1, Saturation1/1
  Ve/1 -> ||V||/1, Demux2/1
  Mux/1 -> asin(vz/Ve)/1
  asin(vz/Ve)/1 -> gammak/1
  Saturation1/1 -> Mux/1
  Demux2/1 -> Terminator2/1
  Demux2/3 -> Mux/2  "vz"
  Demux2/2 -> Terminator1/1

== system Miss_Sim_MatrixPilot/Aerodynamics &  Equations of Motion/Thrust Model ==
  Va : Inport
  Thrust : Inport  Port=2
  0  10000 : Saturate  UpperLimit=10000  LowerLimit=0  OutDataType=sfix(16)  OutScaling=2^0
  Gain1 : Gain  Gain=Tmax  SaturateOnIntegerOverflow=on
  Gain2 : Gain  Gain=Tmax/Vmax  SaturateOnIntegerOverflow=on
  Mass1 : Constant  Value=0
  Mass2 : Constant  Value=0
  Mux2 : Mux  Inputs=3
  Sum1 : Sum  Inputs=+-  InputSameDT=on
  Thrust Model : Scope  NumInputPorts=3
      settings: TimeRange=20  YMin=-1~-20~-1  YMax=1~5~1  SaveName=ScopeData19  MaxDataPoints=600000  Decimation=10  SampleInput=on
  F : Outport
  wires:
  Thrust/1 -> Gain1/1, Thrust Model/1  "Thrust"
  Mux2/1 -> F/1
  Mass2/1 -> Mux2/2
  Mass1/1 -> Mux2/3
  Gain1/1 -> Sum1/1
  Sum1/1 -> 0  10000/1
  Va/1 -> Gain2/1, Thrust Model/2  "Va"
  Gain2/1 -> Sum1/2
  0  10000/1 -> Mux2/1, Thrust Model/3

== system Miss_Sim_MatrixPilot/Aerodynamics &  Equations of Motion/Weight Model ==
  Euler : Inport
  " Function" : Trigonometry
  " Function1" : Trigonometry  Operator=cos
  " Function2" : Trigonometry
  " Function3" : Trigonometry  Operator=cos
  Demux1 : Demux  Outputs=3
  Gain : Gain  Gain=9.81  SaturateOnIntegerOverflow=on
  Gain1 : Gain  Gain=-1  SaturateOnIntegerOverflow=on
  Mass : Constant  Value=Mass
  Mux2 : Mux  Inputs=3
  Product : Product  SaturateOnIntegerOverflow=on  RndMeth=Zero  InputSameDT=on
  Product1 : Product  SaturateOnIntegerOverflow=on  RndMeth=Zero  InputSameDT=on
  Product2 : Product  SaturateOnIntegerOverflow=on  RndMeth=Zero  InputSameDT=on
  Terminator : Terminator
  Weight : Outport
  wires:
  Euler/1 -> Demux1/1
  Demux1/2 -> " Function"/1, " Function1"/1  "theta"
  Mass/1 -> Gain/1
  Mux2/1 -> Product/2
  Product/1 -> Weight/1
  Gain/1 -> Product/1
  " Function"/1 -> Gain1/1
  " Function1"/1 -> Product2/2, Product1/1
  Demux1/1 -> " Function2"/1, " Function3"/1  "phi"
  " Function2"/1 -> Product2/1
  Product2/1 -> Mux2/2
  Gain1/1 -> Mux2/1
  " Function3"/1 -> Product1/2
  Product1/1 -> Mux2/3
  Demux1/3 -> Terminator/1  "psi"

== system Miss_Sim_MatrixPilot/Systems/Actuators ==
  rudc : Inport
  elec : Inport  Port=2
  Tc : Inport  Port=3
  Actuators : Scope  NumInputPorts=3
      settings: TimeRange=90  YMin=-30~-30~0  YMax=30~30~1  SaveName=ScopeData26  MaxDataPoints=6000000  Decimation=10  SampleInput=on
  BEC : simulink_extras/Additional Linear/Transfer Fcn (with initial states)  SystemSampleTime=-1  N=[1]  D="[0.03  1]"  X0=0
  Elevator servo+fin : Subsystem  mask(Second Order Nonlinear Actuator){wn=ele_frequency, z=ele_damping, def_max=ele_def_max, def_max_rate=ele_rate_limit, def_0=0}
      mask prompts: wn "Natural frequency"; z "Damping ratio"; def_max "Deflection limit"; def_max_rate "Rate limit"; def_0 "Initial position"
      mask help: Implement a second-order actuator model with saturation and rate limits.
  Mux : Mux  Inputs=3
  Mux1 : Mux  Inputs=2
  Mux2 : Mux  Inputs=2
  Rho6 : Constant  Value=0
  Rudder servo+fin : Subsystem  mask(Second Order Nonlinear Actuator){wn=rud_frequency, z=rud_damping, def_max=rud_def_max, def_max_rate=rud_rate_limit, def_0=0}
      mask prompts: wn "Natural frequency"; z "Damping ratio"; def_max "Deflection limit"; def_max_rate "Rate limit"; def_0 "Initial position"
      mask help: Implement a second-order actuator model with saturation and rate limits.
  Control surfaces : Outport
  Thrust : Outport  Port=2
  wires:
  Mux/1 -> Control surfaces/1
  Elevator servo+fin/1(Deflec) -> Mux1/2, Mux/2  "ele"
  Rho6/1 -> Mux/1
  rudc/1 -> Mux2/1, Rudder servo+fin/1(Cmd deflec)  "rudc"
  Tc/1 -> BEC/1  "Tc"
  BEC/1 -> Thrust/1, Actuators/3  "Thrust"
  Rudder servo+fin/1(Deflec) -> Mux/3, Mux2/2  "rud"
  elec/1 -> Mux1/1, Elevator servo+fin/1(Cmd deflec)  "elec"
  Mux2/1 -> Actuators/1
  Mux1/1 -> Actuators/2

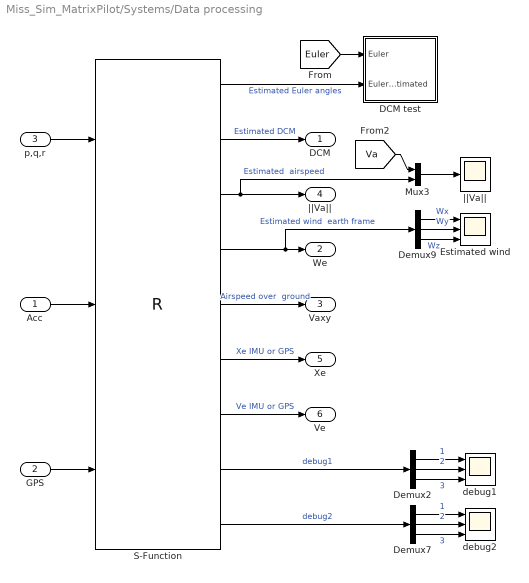
== system Miss_Sim_MatrixPilot/Systems/Data processing ==
  Acc : Inport
  GPS : Inport  Port=2
  p,q,r : Inport  Port=3
  DCM test : Subsystem
  Demux2 : Demux  Outputs=3
  Demux7 : Demux  Outputs=3
  Demux9 : Demux  Outputs=3
  Estimated wind : Scope  NumInputPorts=3
      settings: TimeRange=1000  YMin=-10~-5~-5  YMax=0~5~5  SaveName=ScopeData12  MaxDataPoints=600000  Decimation=100
  Mux3 : Mux  Inputs=2
  S-Function : S-Function  FunctionName=R  Parameters=Rpar
  debug1 : Scope  NumInputPorts=3
      settings: TimeRange=20  YMin=-1~-20~-1  YMax=1~5~1  SaveName=ScopeData28  MaxDataPoints=600000  Decimation=10  SampleInput=on
  debug2 : Scope  NumInputPorts=3
      settings: TimeRange=180  YMin=-10~-1~0  YMax=27.5~6~60  SaveName=ScopeData27  MaxDataPoints=600000  Decimation=10  SampleInput=on
  "||Va|| " : Scope
      settings: TimeRange=1000  YMin=0  YMax=12  SaveName=ScopeData31  MaxDataPoints=600000  Decimation=10
  DCM : Outport
  We : Outport  Port=2
  Vaxy : Outport  Port=3
  ||Va|| : Outport  Port=4
  Xe : Outport  Port=5
  Ve : Outport  Port=6
  wires:
  S-Function/1 -> DCM test/2(Euler estimated)  "Estimated Euler angles"
  S-Function/3 -> ||Va||/1, Mux3/2  "Estimated  airspeed"
  S-Function/2 -> DCM/1  "Estimated DCM"
  p,q,r/1 -> S-Function/1
  Acc/1 -> S-Function/2
  GPS/1 -> S-Function/3
  [Euler] -> DCM test/1(Euler)
  S-Function/5 -> Vaxy/1  "Airspeed over  ground"
  S-Function/4 -> We/1, Demux9/1  "Estimated wind  earth frame"
  Demux9/1 -> Estimated wind/1  "Wx"
  Demux9/2 -> Estimated wind/2  "Wy"
  Demux9/3 -> Estimated wind/3  "Wz"
  S-Function/8 -> Demux2/1  "debug1"
  S-Function/7 -> Ve/1  "Ve IMU or GPS"
  S-Function/6 -> Xe/1  "Xe IMU or GPS"
  Demux2/1 -> debug1/1  "1"
  Demux2/2 -> debug1/2  "2"
  Demux7/2 -> debug2/2  "2"
  Demux7/1 -> debug2/1  "1"
  S-Function/9 -> Demux7/1  "debug2"
  Demux2/3 -> debug1/3  "3"
  Demux7/3 -> debug2/3  "3"
  Mux3/1 -> "||Va|| "/1
  [Va] -> Mux3/1

== system Miss_Sim_MatrixPilot/Systems/NGC ==
  DCM : Inport
  We : Inport  Port=2
  Vaxy : Inport  Port=3
  ||Va|| : Inport  Port=4
  Xe : Inport  Port=5
  Ve : Inport  Port=6
  p,q,r : Inport  Port=7
  Control : Subsystem  TreatAsAtomicUnit=on  SystemSampleTime=0.025
  Guidance : Subsystem  TreatAsAtomicUnit=on  SystemSampleTime=0.025
  Navigation : Subsystem  TreatAsAtomicUnit=on  SystemSampleTime=0.025
  rudc : Outport
  elec : Outport  Port=2
  Tc : Outport  Port=3
  wires:
  Guidance/3(thetac) -> Control/2(thetac)
  p,q,r/1 -> Control/4(p,q,r)
  ||Va||/1 -> Guidance/5(||Va||)
  Navigation/2(zec) -> Guidance/2(zec)
  Guidance/1(Tc) -> Tc/1
  Guidance/2(yawc) -> Control/1(yawc)
  Navigation/1(psic) -> Guidance/1(psic)
  Control/1(rudc) -> rudc/1
  Control/2(elec) -> elec/1
  DCM/1 -> Guidance/6(DCM), Control/3(DCM)
  We/1 -> Navigation/1(We)
  Vaxy/1 -> Navigation/2(Vaxy)
  Xe/1 -> Navigation/3(Xe), Guidance/3(Xe)
  Ve/1 -> Guidance/4(Ve)

== system Miss_Sim_MatrixPilot/Systems/Sensors ==
  p,q,r : Inport
  Ab : Inport  Port=2
  Euler : Inport  Port=3
  Ve : Inport  Port=4
  Xe : Inport  Port=5
  Accelerometers : Subsystem
  EM-406 GPS : Subsystem
  Gyros : Subsystem
  Acc : Outport
  GPS : Outport  Port=2
  "p,q,r " : Outport  Port=3
  wires:
  Gyros/1("p,q,r ") -> "p,q,r "/1
  Ve/1 -> EM-406 GPS/1(Ve)
  p,q,r/1 -> Gyros/1(p,q,r)
  Ab/1 -> Accelerometers/1(Ab)
  Euler/1 -> Accelerometers/2(Euler)
  Accelerometers/1(Acc) -> Acc/1
  Xe/1 -> EM-406 GPS/2(Xe)
  EM-406 GPS/1(GPS) -> GPS/1

== system Miss_Sim_MatrixPilot/Wind/Wind custom ==
  DCM : Inport
  Speed : Inport  Port=2
  Direction (°) : Inport  Port=3
  Wez : Inport  Port=4
  Degrees to Radians : simulink_extras/Transformations/Degrees to Radians  SystemSampleTime=-1
  Mux : Mux  Inputs=3
  Prodct2 : Product  Multiplication=Matrix(*)  SaturateOnIntegerOverflow=on  RndMeth=Zero  InputSameDT=on
  Product : Product  OutDataType=sfix(16)  OutScaling=2^0  RndMeth=Zero
  Product1 : Product  OutDataType=sfix(16)  OutScaling=2^0  RndMeth=Zero
  Trigonometric Function : Trigonometry  Operator=cos
  Trigonometric Function1 : Trigonometry
  Wb : Outport
  wires:
  Wez/1 -> Mux/3  "Wez"
  Direction (°)/1 -> Degrees to Radians/1
  Trigonometric Function/1 -> Product/2
  Trigonometric Function1/1 -> Product1/2
  Speed/1 -> Product1/1, Product/1
  Product1/1 -> Mux/2  "Wey"
  Product/1 -> Mux/1  "Wex"
  DCM/1 -> Prodct2/1
  Mux/1 -> Prodct2/2  "We"
  Prodct2/1 -> Wb/1
  Degrees to Radians/1 -> Trigonometric Function/1, Trigonometric Function1/1

== system Miss_Sim_MatrixPilot/Systems/Actuators/Elevator servo+fin ==
  Cmd deflec : Inport  OutDataType=sfix(16)  OutScaling=2^0
  2*zeta * wn : Gain  Orientation=left  Gain=2.* z*wn  ParameterDataType=sfix(16)  ParameterScaling=2^0  OutDataType=sfix(16)  OutScaling=2^0  SaturateOnIntegerOverflow=on
  Degrees to Radians : simulink_extras/Transformations/Degrees to Radians  SystemSampleTime=-1
  Demand limits : Saturate  UpperLimit=def_max  LowerLimit=-def_max
  Limited Deflection : Integrator  InitialCondition=def_0  LimitOutput=on  UpperSaturationLimit=def_max  LowerSaturationLimit=-def_max
  Radians to Degrees : simulink_extras/Transformations/Radians to Degrees  SystemSampleTime=-1
  Servo rate : Integrator
  Sum2 : Sum  Inputs=|+-  OutDataType=sfix(16)  OutScaling=2^0  SaturateOnIntegerOverflow=on  InputSameDT=on
  Sum3 : Sum  Inputs=|+-  OutDataType=sfix(16)  OutScaling=2^0  SaturateOnIntegerOverflow=on  InputSameDT=on
  rate limit*2*zeta/wn : Saturate  UpperLimit=def_max_rate*2*z/wn  LowerLimit=-def_max_rate*2*z/wn
  wn^2 : Gain  Gain=wn*wn  ParameterDataType=sfix(16)  ParameterScaling=2^0  OutDataType=sfix(16)  OutScaling=2^0  SaturateOnIntegerOverflow=on
  Deflec : Outport  OutDataType=sfix(16)  OutScaling=2^0  InitialOutput=0
  wires:
  Cmd deflec/1 -> Degrees to Radians/1
  Demand limits/1 -> Sum3/1
  rate limit*2*zeta/wn/1 -> wn^2/1
  Sum3/1 -> rate limit*2*zeta/wn/1
  2*zeta * wn/1 -> Sum2/2
  Servo rate/1 -> Limited Deflection/1, 2*zeta * wn/1
  Sum2/1 -> Servo rate/1
  wn^2/1 -> Sum2/1
  Limited Deflection/1 -> Sum3/2, Radians to Degrees/1
  Radians to Degrees/1 -> Deflec/1
  Degrees to Radians/1 -> Demand limits/1

== system Miss_Sim_MatrixPilot/Systems/Actuators/Rudder servo+fin ==
  Cmd deflec : Inport  OutDataType=sfix(16)  OutScaling=2^0
  2*zeta * wn : Gain  Orientation=left  Gain=2.* z*wn  ParameterDataType=sfix(16)  ParameterScaling=2^0  OutDataType=sfix(16)  OutScaling=2^0  SaturateOnIntegerOverflow=on
  Degrees to Radians : simulink_extras/Transformations/Degrees to Radians  SystemSampleTime=-1
  Demand limits : Saturate  UpperLimit=def_max  LowerLimit=-def_max
  Limited Deflection : Integrator  InitialCondition=def_0  LimitOutput=on  UpperSaturationLimit=def_max  LowerSaturationLimit=-def_max
  Radians to Degrees : simulink_extras/Transformations/Radians to Degrees  SystemSampleTime=-1
  Servo rate : Integrator
  Sum2 : Sum  Inputs=|+-  OutDataType=sfix(16)  OutScaling=2^0  SaturateOnIntegerOverflow=on  InputSameDT=on
  Sum3 : Sum  Inputs=|+-  OutDataType=sfix(16)  OutScaling=2^0  SaturateOnIntegerOverflow=on  InputSameDT=on
  rate limit*2*zeta/wn : Saturate  UpperLimit=def_max_rate*2*z/wn  LowerLimit=-def_max_rate*2*z/wn
  wn^2 : Gain  Gain=wn*wn  ParameterDataType=sfix(16)  ParameterScaling=2^0  OutDataType=sfix(16)  OutScaling=2^0  SaturateOnIntegerOverflow=on
  Deflec : Outport  OutDataType=sfix(16)  OutScaling=2^0  InitialOutput=0
  wires:
  Cmd deflec/1 -> Degrees to Radians/1
  Demand limits/1 -> Sum3/1
  rate limit*2*zeta/wn/1 -> wn^2/1
  Sum3/1 -> rate limit*2*zeta/wn/1
  2*zeta * wn/1 -> Sum2/2
  Servo rate/1 -> Limited Deflection/1, 2*zeta * wn/1
  Sum2/1 -> Servo rate/1
  wn^2/1 -> Sum2/1
  Limited Deflection/1 -> Sum3/2, Radians to Degrees/1
  Radians to Degrees/1 -> Deflec/1
  Degrees to Radians/1 -> Demand limits/1

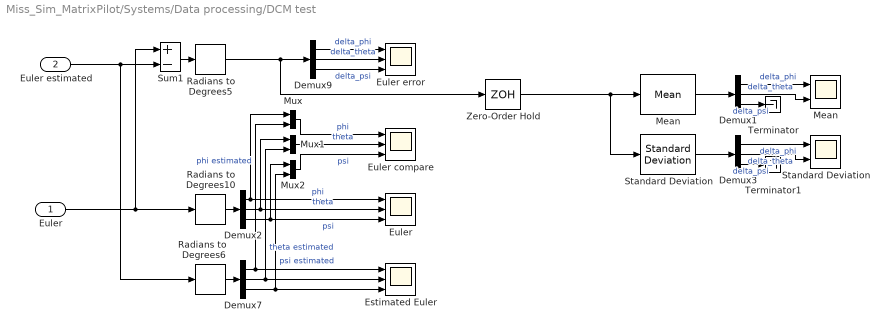
== system Miss_Sim_MatrixPilot/Systems/Data processing/DCM test ==
  Euler : Inport
  Euler estimated : Inport  Port=2
  Demux{1..3,7,9} (5 alike) : Demux  Outputs=3
  Estimated Euler : Scope  NumInputPorts=3
      settings: TimeRange=180  YMin=-10~-1~0  YMax=27.5~6~60  SaveName=ScopeData22  MaxDataPoints=600000  Decimation=10  SampleInput=on
  "Euler  " : Scope  NumInputPorts=3
      settings: TimeRange=20  YMin=-1~-20~-1  YMax=1~5~1  SaveName=ScopeData25  MaxDataPoints=600000  Decimation=10  SampleInput=on
  Euler compare : Scope  NumInputPorts=3
      settings: TimeRange=300  YMin=-50~-30~-200  YMax=50~20~200  SaveName=ScopeData23  MaxDataPoints=600000  Decimation=10
  Euler error : Scope  NumInputPorts=3
      settings: TimeRange=50  YMin=-1~1.1~-1  YMax=1~2.4~1  SaveName=ScopeData24  MaxDataPoints=600000  Decimation=10
  Mean : dspstat3/Mean  DialogController=dspDDGCreate  DialogControllerArgs=DataTag0  run=on  reset_popup=None  roundingMode=Floor  overflowMode=off
  "Mean " : Scope  NumInputPorts=2
      settings: TimeRange=300  YMin=-0.5~-3  YMax=1.5~3  SaveName=ScopeData20  MaxDataPoints=600000  Decimation=10
  Mux : Mux  Inputs=2
  Mux1 : Mux  Inputs=2
  Mux2 : Mux  Inputs=2
  Radians to Degrees10 : simulink_extras/Transformations/Radians to Degrees  SystemSampleTime=-1
  Radians to Degrees5 : simulink_extras/Transformations/Radians to Degrees  SystemSampleTime=-1
  Radians to Degrees6 : simulink_extras/Transformations/Radians to Degrees  SystemSampleTime=-1
  Standard Deviation : dspstat3/Standard Deviation  run=on  reset_popup=None
  "Standard Deviation " : Scope  NumInputPorts=2
      settings: TimeRange=600  YMin=0.72~0.905  YMax=0.775~0.965  SaveName=ScopeData30  MaxDataPoints=600000  Decimation=10
  Sum1 : Sum  Inputs=+-  SaturateOnIntegerOverflow=on  InputSameDT=on
  Terminator : Terminator
  Terminator1 : Terminator
  Zero-Order Hold : ZeroOrderHold  SampleTime=0.0005
  wires:
  Demux2/1 -> "Euler  "/1, Mux/1  "phi"
  Demux2/2 -> "Euler  "/2, Mux1/1  "theta"
  Euler/1 -> Sum1/1, Radians to Degrees10/1
  Demux7/2 -> Estimated Euler/2, Mux1/2  "theta estimated"
  Demux7/1 -> Estimated Euler/1, Mux/2  "phi estimated"
  Radians to Degrees6/1 -> Demux7/1
  Sum1/1 -> Radians to Degrees5/1
  Demux9/1 -> Euler error/1  "delta_phi"
  Demux9/2 -> Euler error/2  "delta_theta"
  Demux9/3 -> Euler error/3  "delta_psi"
  Radians to Degrees5/1 -> Demux9/1, Zero-Order Hold/1
  Demux2/3 -> "Euler  "/3, Mux2/1  "psi"
  Demux7/3 -> Estimated Euler/3, Mux2/2  "psi estimated"
  Mux/1 -> Euler compare/1  "phi"
  Mux1/1 -> Euler compare/2  "theta"
  Mux2/1 -> Euler compare/3  "psi"
  Radians to Degrees10/1 -> Demux2/1
  Euler estimated/1 -> Radians to Degrees6/1, Sum1/2
  Demux1/1 -> "Mean "/1  "delta_phi"
  Demux1/2 -> "Mean "/2  "delta_theta"
  Demux3/1 -> "Standard Deviation "/1  "delta_phi"
  Demux3/2 -> "Standard Deviation "/2  "delta_theta"
  Mean/1 -> Demux1/1
  Standard Deviation/1 -> Demux3/1
  Zero-Order Hold/1 -> Mean/1, Standard Deviation/1
  Demux1/3 -> Terminator/1  "delta_psi"
  Demux3/3 -> Terminator1/1  "delta_psi"

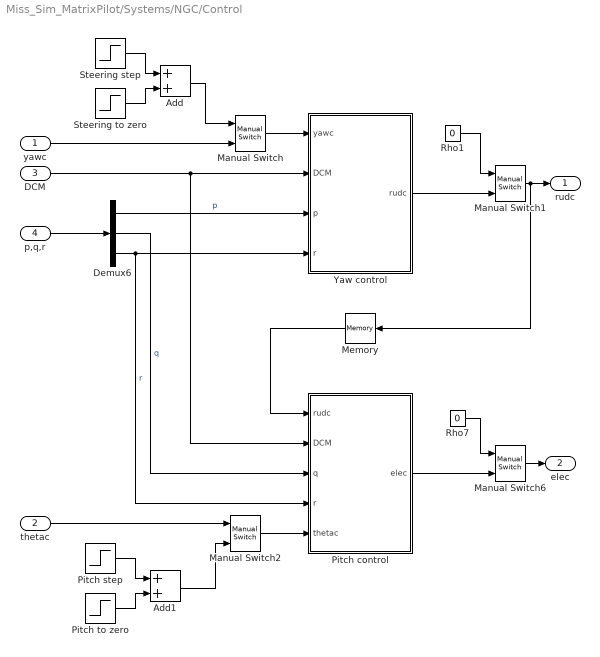
== system Miss_Sim_MatrixPilot/Systems/NGC/Control ==
  yawc : Inport
  thetac : Inport  Port=2
  DCM : Inport  Port=3
  p,q,r : Inport  Port=4
  Add : Sum  OutDataType=sfix(16)  OutScaling=2^-10
  Add1 : Sum  OutDataType=sfix(16)  OutScaling=2^-10
  Demux6 : Demux  Outputs=3
  Manual Switch : simulink/Signal Routing/Manual Switch  SystemSampleTime=-1  sw=0  action=0  varsize=off
  Manual Switch1 : simulink/Signal Routing/Manual Switch  SystemSampleTime=-1  sw=0  action=0  varsize=off
  Manual Switch2 : simulink/Signal Routing/Manual Switch  SystemSampleTime=-1  sw=1  action=0  varsize=off
  Manual Switch6 : simulink/Signal Routing/Manual Switch  SystemSampleTime=-1  sw=0  action=0  varsize=off
  Memory : Memory  Orientation=left  InheritSampleTime=on
  Pitch control : Subsystem
  Pitch step : Step  Time=5  After=20
  Pitch to zero : Step  Time=10  After=-20
  Rho1 : Constant  Value=0
  Rho7 : Constant  Value=0
  Steering step : Step  Time=5  After=30/180*pi()
  Steering to zero : Step  Time=10  After=-30/180*pi()
  Yaw control : Subsystem
  rudc : Outport
  elec : Outport  Port=2
  wires:
  p,q,r/1 -> Demux6/1
  Demux6/2 -> Pitch control/3(q)  "q"
  Pitch control/1(elec) -> Manual Switch6/2
  Manual Switch6/1 -> elec/1
  Rho7/1 -> Manual Switch6/1
  Demux6/1 -> Yaw control/3(p)  "p"
  Demux6/3 -> Yaw control/4(r), Pitch control/4(r)  "r"
  Memory/1 -> Pitch control/1(rudc)
  DCM/1 -> Yaw control/2(DCM), Pitch control/2(DCM)
  Manual Switch/1 -> Yaw control/1(yawc)
  yawc/1 -> Manual Switch/2
  Steering step/1 -> Add/1
  Steering to zero/1 -> Add/2
  Add/1 -> Manual Switch/1
  Rho1/1 -> Manual Switch1/1
  Yaw control/1(rudc) -> Manual Switch1/2
  Manual Switch1/1 -> rudc/1, Memory/1
  Pitch step/1 -> Add1/1
  Pitch to zero/1 -> Add1/2
  Add1/1 -> Manual Switch2/2
  Manual Switch2/1 -> Pitch control/5(thetac)
  thetac/1 -> Manual Switch2/1

== system Miss_Sim_MatrixPilot/Systems/NGC/Guidance ==
  psic : Inport
  zec : Inport  Port=2
  Xe : Inport  Port=3
  Ve : Inport  Port=4
  ||Va|| : Inport  Port=5
  DCM : Inport  Port=6
  Altitude control : Subsystem  SystemSampleTime=0.025
  Heading step : Step  Time=5  After=pi()/2
  Heading control : Subsystem  SystemSampleTime=0.025
  Manual Switch : simulink/Signal Routing/Manual Switch  SystemSampleTime=-1  sw=0  action=0  varsize=off
  Manual Switch1 : simulink/Signal Routing/Manual Switch  SystemSampleTime=-1  sw=0  action=0  varsize=off
  Manual Switch9 : simulink/Signal Routing/Manual Switch  SystemSampleTime=-1  sw=0  action=0  varsize=off
  Rho1 : Constant  Value=0.7
  Rho2 : Constant  Value=0
  Selector2 : Selector  InputPortWidth=3  IndexOptions=Index vector (dialog)  Indices=[3]  OutputSizes=1
  Tc : Outport
  yawc : Outport  Port=2
  thetac : Outport  Port=3
  wires:
  Xe/1 -> Selector2/1
  zec/1 -> Altitude control/1(zec)
  Heading control/1(yawc) -> yawc/1
  Manual Switch9/1 -> thetac/1
  Altitude control/1(thetac) -> Manual Switch9/2
  Rho2/1 -> Manual Switch9/1
  ||Va||/1 -> Altitude control/3(||Va||)
  Ve/1 -> Altitude control/4(Ve)
  Manual Switch1/1 -> Tc/1
  Rho1/1 -> Manual Switch1/1
  Altitude control/2(Tc) -> Manual Switch1/2
  Selector2/1 -> Altitude control/2(ze)  "ze"
  DCM/1 -> Heading control/2(DCM)
  Manual Switch/1 -> Heading control/1(psic)
  psic/1 -> Manual Switch/2
  Heading step/1 -> Manual Switch/1

== system Miss_Sim_MatrixPilot/Systems/NGC/Navigation ==
  We : Inport
  Vaxy : Inport  Port=2
  Xe : Inport  Port=3
  Degrees to Radians : simulink_extras/Transformations/Degrees to Radians  SystemSampleTime=-1
  Embedded MATLAB Function : Stateflow chart
  KPZ1 : Gain  Gain=-1  SaturateOnIntegerOverflow=on
  Manual Switch1 : simulink/Signal Routing/Manual Switch  SystemSampleTime=-1  sw=1  action=0  varsize=off
  Manual Switch2 : simulink/Signal Routing/Manual Switch  SystemSampleTime=-1  sw=0  action=0  varsize=off
  Manual Switch3 : simulink/Signal Routing/Manual Switch  SystemSampleTime=-1  sw=0  action=0  varsize=off
  Navigation : Scope  NumInputPorts=2
      settings: TimeRange=10  YMin=2.3~-50.5  YMax=3.2~-49.8  SaveName=ScopeData21  MaxDataPoints=600000  Decimation=10
  Radians to Degrees6 : simulink_extras/Transformations/Radians to Degrees  SystemSampleTime=-1
  Rho1 : Constant  Value=0
  Rho2 : Constant  Value=0
  Rho3 : Constant  Value=CROSS_TRACK
  Rho4 : Constant  Value=WAYPOINT_RADIUS
  Rho5 : Constant  Value=-75
  Sum2 : Sum  SaturateOnIntegerOverflow=on  InputSameDT=on
  debug : Scope
      settings: TimeRange=30  YMin=-25  YMax=15  SaveName=ScopeData17  MaxDataPoints=600000  Decimation=10
  psic : Outport
  zec : Outport  Port=2
  wires:
  Rho1/1 -> Degrees to Radians/1
  Rho5/1 -> Manual Switch1/1, Sum2/1  "Hc"
  Manual Switch1/1 -> Manual Switch2/1
  Manual Switch3/1 -> psic/1
  Rho2/1 -> KPZ1/1
  KPZ1/1 -> Sum2/2
  Sum2/1 -> Manual Switch1/2
  Manual Switch2/1 -> zec/1
  Embedded MATLAB Function/2(psic) -> Manual Switch3/2, Radians to Degrees6/1
  Embedded MATLAB Function/3(zec) -> Manual Switch2/2, Navigation/1
  Embedded MATLAB Function/1(debug) -> debug/1
  Xe/1 -> Embedded MATLAB Function/5(Xe)
  Vaxy/1 -> Embedded MATLAB Function/4(Vaxy)
  We/1 -> Embedded MATLAB Function/3(We)
  Rho3/1 -> Embedded MATLAB Function/1(CROSS_TRACK)
  Rho4/1 -> Embedded MATLAB Function/2(WAYPOINT_RADIUS)
  Radians to Degrees6/1 -> Navigation/2
  Degrees to Radians/1 -> Manual Switch3/1

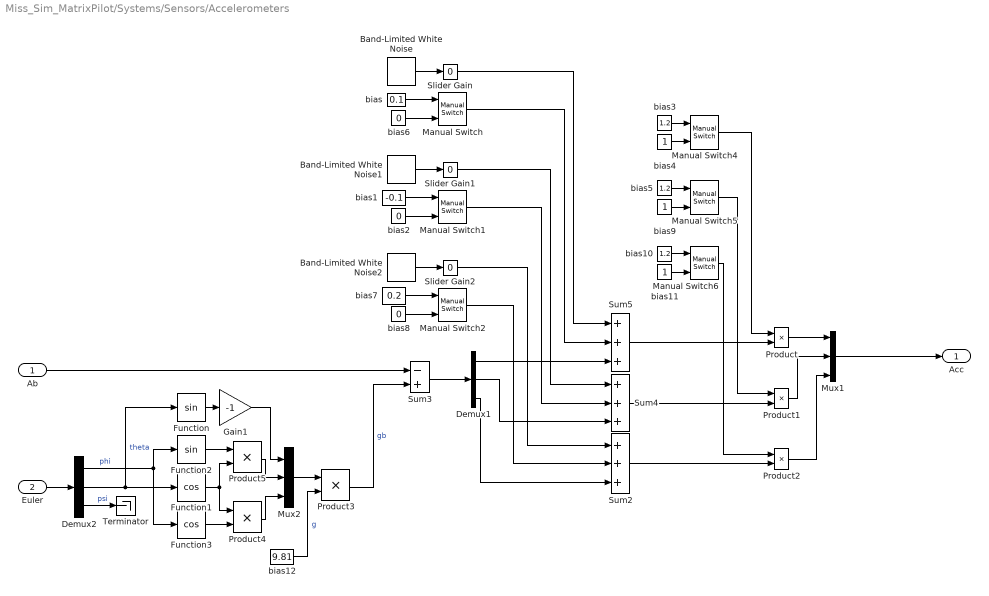
== system Miss_Sim_MatrixPilot/Systems/Sensors/Accelerometers ==
  Ab : Inport
  Euler : Inport  Port=2
  " Function" : Trigonometry
  " Function1" : Trigonometry  Operator=cos
  " Function2" : Trigonometry
  " Function3" : Trigonometry  Operator=cos
  Band-Limited White Noise : simulink/Sources/Band-Limited White Noise  SystemSampleTime=-1  Cov=[0.000001]  Ts=0.01  seed=[23341]
  Band-Limited White Noise1 : simulink/Sources/Band-Limited White Noise  SystemSampleTime=-1  Cov=[0.000001]  Ts=0.01  seed=[23341]
  Band-Limited White Noise2 : simulink/Sources/Band-Limited White Noise  SystemSampleTime=-1  Cov=[0.000001]  Ts=0.01  seed=[23341]
  Demux1 : Demux  Outputs=3
  Demux2 : Demux  Outputs=3
  Gain1 : Gain  Gain=-1  SaturateOnIntegerOverflow=on
  Manual Switch{,1..2,4..6} (6 alike) : simulink/Signal Routing/Manual Switch  SystemSampleTime=-1  sw=0  action=0  varsize=off
  Mux1 : Mux  Inputs=3
  Mux2 : Mux  Inputs=3
  Product{,1..5} (6 alike) : Product  SaturateOnIntegerOverflow=on  RndMeth=Zero  InputSameDT=on
  Slider Gain : simulink/Math Operations/Slider Gain  SystemSampleTime=-1  low=0  gain=0  high=2
  Slider Gain1 : simulink/Math Operations/Slider Gain  SystemSampleTime=-1  low=0  gain=0  high=2
  Slider Gain2 : simulink/Math Operations/Slider Gain  SystemSampleTime=-1  low=0  gain=0  high=2
  Sum2 : Sum  Inputs=+++  SaturateOnIntegerOverflow=on  InputSameDT=on
  Sum3 : Sum  Inputs=-+  SaturateOnIntegerOverflow=on  InputSameDT=on
  Sum4 : Sum  Inputs=+++  SaturateOnIntegerOverflow=on  InputSameDT=on
  Sum5 : Sum  Inputs=+++  SaturateOnIntegerOverflow=on  InputSameDT=on
  Terminator : Terminator
  bias : Constant  Value=0.1  VectorParams1D=off
  bias1 : Constant  Value=-0.1  VectorParams1D=off
  bias10 : Constant  Value=1.2  VectorParams1D=off
  bias11 : Constant  VectorParams1D=off
  bias12 : Constant  Value=9.81  VectorParams1D=off
  bias2 : Constant  Value=0  VectorParams1D=off
  bias3 : Constant  Value=1.2  VectorParams1D=off
  bias4 : Constant  VectorParams1D=off
  bias5 : Constant  Value=1.2  VectorParams1D=off
  bias6 : Constant  Value=0  VectorParams1D=off
  bias7 : Constant  Value=0.2  VectorParams1D=off
  bias8 : Constant  Value=0  VectorParams1D=off
  bias9 : Constant  VectorParams1D=off
  Acc : Outport
  wires:
  Mux1/1 -> Acc/1
  Band-Limited White Noise/1 -> Slider Gain/1
  Demux1/3 -> Sum2/3
  Demux1/2 -> Sum4/3
  Demux1/1 -> Sum5/3
  Band-Limited White Noise1/1 -> Slider Gain1/1
  Band-Limited White Noise2/1 -> Slider Gain2/1
  Slider Gain2/1 -> Sum2/1
  Slider Gain1/1 -> Sum4/1
  Slider Gain/1 -> Sum5/1
  Sum5/1 -> Product/2
  Product/1 -> Mux1/1
  Sum4/1 -> Product1/2
  Product1/1 -> Mux1/2
  Sum2/1 -> Product2/2
  Product2/1 -> Mux1/3
  Manual Switch4/1 -> Product/1
  Manual Switch6/1 -> Product2/1
  Manual Switch5/1 -> Product1/1
  Manual Switch/1 -> Sum5/2
  bias/1 -> Manual Switch/1
  bias6/1 -> Manual Switch/2
  bias1/1 -> Manual Switch1/1
  bias2/1 -> Manual Switch1/2
  bias7/1 -> Manual Switch2/1
  bias8/1 -> Manual Switch2/2
  Manual Switch2/1 -> Sum2/2
  Manual Switch1/1 -> Sum4/2
  bias3/1 -> Manual Switch4/1
  bias4/1 -> Manual Switch4/2
  bias5/1 -> Manual Switch5/1
  bias9/1 -> Manual Switch5/2
  bias10/1 -> Manual Switch6/1
  bias11/1 -> Manual Switch6/2
  Sum3/1 -> Demux1/1
  Ab/1 -> Sum3/1
  Euler/1 -> Demux2/1
  Demux2/2 -> " Function"/1, " Function1"/1  "theta"
  " Function"/1 -> Gain1/1
  " Function1"/1 -> Product5/2, Product4/1
  Demux2/1 -> " Function2"/1, " Function3"/1  "phi"
  " Function2"/1 -> Product5/1
  Product5/1 -> Mux2/2
  Gain1/1 -> Mux2/1
  " Function3"/1 -> Product4/2
  Product4/1 -> Mux2/3
  Demux2/3 -> Terminator/1  "psi"
  Mux2/1 -> Product3/1
  bias12/1 -> Product3/2  "g"
  Product3/1 -> Sum3/2  "gb"
